simulink model "opti_ext"  (R2020a)
settings: Solver=VariableStepAuto  StartTime=0.0  StopTime=10.0  RelTol=1e-3
values from neighbouring files (symbols this model uses):
  k1 = K(1)    [ISEUfunc.m]    (also in ISEfunc.m; ITSEfunc.m; costMpfunc.m; costTr1_100Mp0func.m)
  k2 = K(2)    [ISEUfunc.m]    (also in ISEfunc.m; ITSEfunc.m; costMpfunc.m; costTr1_100Mp0func.m)
settings Model: Creator=Mertcan  LastModifiedBy=Mertcan

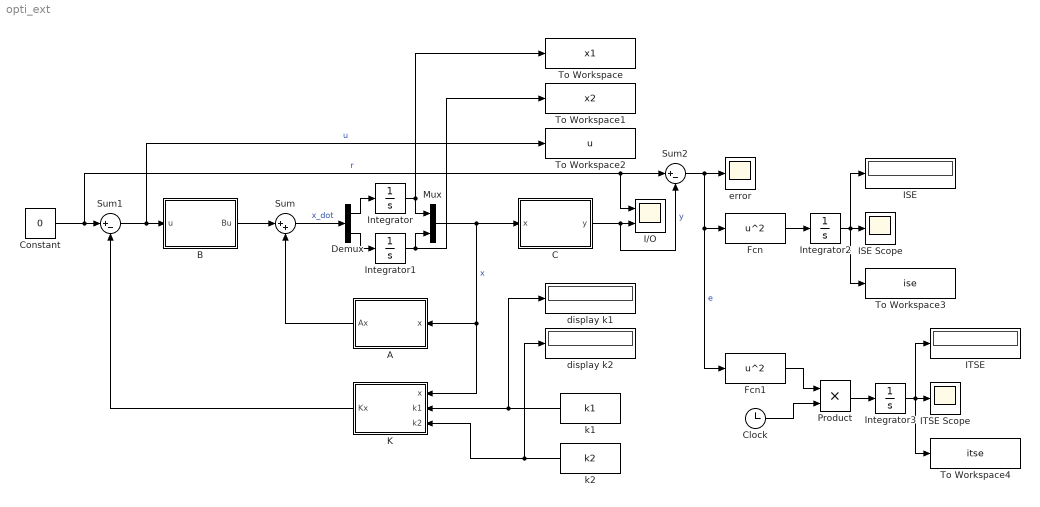
== system opti_ext ==
  A : MATLAB Function  TreatAsAtomicUnit=on
  B : MATLAB Function  TreatAsAtomicUnit=on
  C : MATLAB Function  TreatAsAtomicUnit=on
  Clock : Clock
  Constant : Constant  Value=0
  Demux : Demux  Outputs=2
  Fcn : Fcn  Expr=u^2
  Fcn1 : Fcn  Expr=u^2
  I/O : Scope  NumInputPorts=2
  ISE : Display
  ISE Scope : Scope
  ITSE : Display
  ITSE Scope : Scope
  Integrator : Integrator  InitialCondition=1
  Integrator1 : Integrator  InitialCondition=-1
  Integrator2 : Integrator
  Integrator3 : Integrator
  K : MATLAB Function  TreatAsAtomicUnit=on
  Mux : Mux  Inputs=2
  Product : Product
  Sum : Sum  Inputs=|++
  Sum1 : Sum  Inputs=|+-
  Sum2 : Sum  Inputs=|+-
  To Workspace : ToWorkspace  VariableName=x1  SaveFormat=Timeseries  SampleTime=-1
  To Workspace1 : ToWorkspace  VariableName=x2  SaveFormat=Timeseries  SampleTime=-1
  To Workspace2 : ToWorkspace  VariableName=u  SaveFormat=Timeseries  SampleTime=-1
  To Workspace3 : ToWorkspace  VariableName=ise  SaveFormat=Timeseries  SampleTime=-1
  To Workspace4 : ToWorkspace  VariableName=itse  SaveFormat=Timeseries  SampleTime=-1
  display k1 : Display
  display k2 : Display
  error : Scope
  k1 : Constant  Value=k1
  k2 : Constant  Value=k2
  wires:
  B/1(Bu) -> Sum/1
  Mux/1 -> C/1(x), A/1(x), K/1(x)  "x"
  Sum/1 -> Demux/1  "x_dot"
  A/1(Ax) -> Sum/2
  K/1(Kx) -> Sum1/2
  Demux/1 -> Integrator/1
  Demux/2 -> Integrator1/1
  Integrator1/1 -> To Workspace1/1, Mux/2
  Integrator/1 -> Mux/1, To Workspace/1
  k1/1 -> K/2(k1), display k1/1
  k2/1 -> K/3(k2), display k2/1
  Constant/1 -> I/O/1, Sum2/1, Sum1/1  "r"
  Sum1/1 -> To Workspace2/1, B/1(u)  "u"
  C/1(y) -> I/O/2, Sum2/2  "y"
  Sum2/1 -> Fcn1/1, Fcn/1, error/1  "e"
  Fcn/1 -> Integrator2/1
  Integrator2/1 -> To Workspace3/1, ISE/1, ISE Scope/1
  Fcn1/1 -> Product/1
  Integrator3/1 -> To Workspace4/1, ITSE/1, ITSE Scope/1
  Product/1 -> Integrator3/1
  Clock/1 -> Product/2

== matlab function opti_ext/B ==
  data: u input size=1; Bu output size=2
function Bu = B(u)

Bu = [0;u];

== matlab function opti_ext/K ==
  data: x input size=2; Kx output size=1; k1 input size=1; k2 input size=1
function Kx = K(x,k1,k2)

Kx = k1*x(1) + k2*x(2);

== matlab function opti_ext/C ==
  data: x input size=2; y output size=1
function y = C(x)

C = [1,0];

y = C*x;

== matlab function opti_ext/A ==
  data: x input size=2; Ax output size=2
function Ax = A(x)

Ax = [x(2);-x(1)];
